simulink model "EE514test1"  (Simulink 7.6)
settings: Solver=ode45  StartTime=0.0  StopTime=10.0  RelTol=1e-6
undefined symbols (not defined in the file or in its folder): sigbuilder_block
settings Model: Creator=Nikola  LastModifiedBy=Nikola
settings DebuggingCC: StrictBusMsg=Warning
settings SimEventsCC: propDiagAttribOutput=1  propDiagFcnCallOutput=1  propDiagStatOutput=0

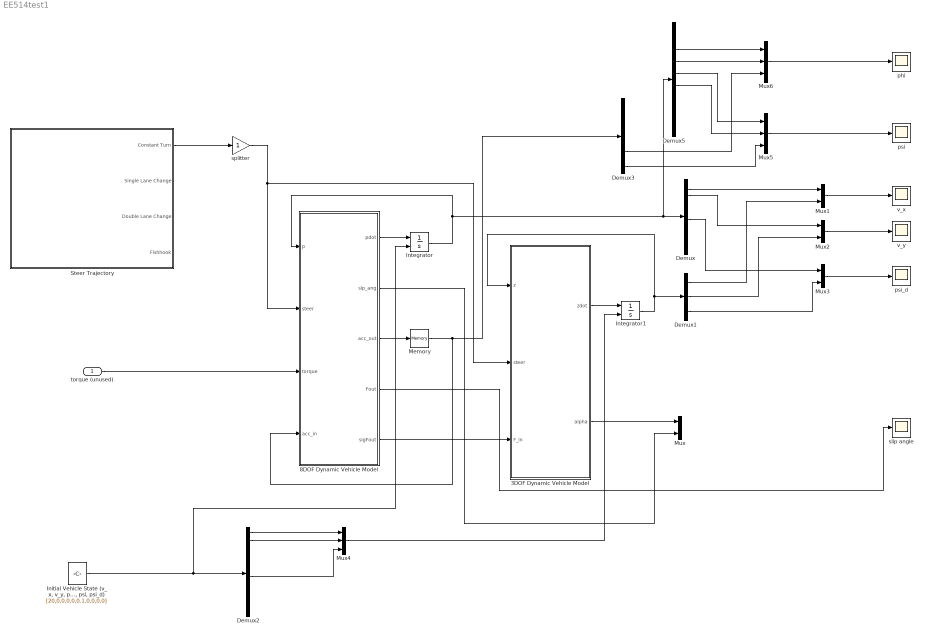
== system EE514test1 ==
  torque (unused) : Inport
  3DOF Dynamic Vehicle Model : Stateflow chart  TreatAsAtomicUnit=on
  8DOF Dynamic Vehicle Model : Stateflow chart  TreatAsAtomicUnit=on
  Demux : Demux  Outputs=10
  Demux1 : Demux  Outputs=3
  Demux2 : Demux  Outputs=10
  Demux3 : Demux  Outputs=5
  Demux5 : Demux  Outputs=10
  "Initial Vehicle State (v_x, v_y, phi, phi_d, psi, psi_d)" : Constant  Value=[20,0,0,0,0,0.1,0,0,0,0]
  Integrator : Integrator  InitialConditionSource=external  InitialCondition=[20,0,0,0,0,0,0,0,0,0]
  Integrator1 : Integrator  InitialConditionSource=external  InitialCondition=[20,0,0]
  Memory : Memory  X0=[0,0,0,0,0]  InheritSampleTime=on
  Mux{,1..3} (4 alike) : Mux  Inputs=2
  Mux4 : Mux  Inputs=3
  Mux5 : Mux  Inputs=3
  Mux6 : Mux  Inputs=3
  Steer Trajectory : Subsystem  Tag=STV Subsys  LoadFcn=sigbuilder_block('load');  StartFcn=sigbuilder_block('start');  StopFcn=sigbuilder_block('stop');  ClipboardFcn=sigbuilder_block('clipboard');  mask(Sigbuilder block){}
      mask help: Create and generate interchangeable groups of signals whose waveforms are piecewise linear.
      mask init:
      | if ~strcmp(get_param(bdroot(gcbh),'SimulationStatus'),'stopped') tuvar = sigbuilder_block('maskInit'); end
      settings: CopyFcn=sigbuilder_block('copy');  DeleteFcn=sigbuilder_block('delete');  ModelCloseFcn=sigbuilder_block('modelClose');  PreSaveFcn=sigbuilder_block('preSave');  NameChangeFcn=sigbuilder_block('namechange');  OpenFcn=sigbuilder_block('open',[-662.25 125.25 479.25 471.75 ]);  CloseFcn=sigbuilder_block('close');
      mask Display: plot(0,0,100,100,[10,10,40,40,10],[80,20,20,80,80],[40,10],[50,50], [40,27,10],[65,72,56],[40,25,25,10],[28,28,43,43]);
  phi : Scope
      settings: SaveName=ScopeData4
  psi : Scope
      settings: SaveName=ScopeData5
  psi_d : Scope
      settings: SaveName=ScopeData3
  slip angle : Scope
  splitter : Gain
  v_x : Scope
  v_y : Scope
      settings: SaveName=ScopeData2
  wires:
  torque (unused)/1 -> 8DOF Dynamic Vehicle Model/3(torque)
  8DOF Dynamic Vehicle Model/3(acc_out) -> Memory/1
  Memory/1 -> 8DOF Dynamic Vehicle Model/4(acc_in), Demux3/1
  8DOF Dynamic Vehicle Model/1(pdot) -> Integrator/1
  3DOF Dynamic Vehicle Model/1(zdot) -> Integrator1/1
  Integrator1/1 -> Demux1/1, 3DOF Dynamic Vehicle Model/1(z)
  splitter/1 -> 3DOF Dynamic Vehicle Model/2(steer), 8DOF Dynamic Vehicle Model/2(steer)
  3DOF Dynamic Vehicle Model/2(alpha) -> Mux/1
  8DOF Dynamic Vehicle Model/2(slp_ang) -> Mux/2
  Demux/1 -> Mux1/1
  Demux/2 -> Mux2/1
  Demux1/2 -> Mux2/2
  Demux/6 -> Mux3/1
  Mux1/1 -> v_x/1
  Mux3/1 -> psi_d/1
  Mux2/1 -> v_y/1
  Demux1/1 -> Mux1/2
  "Initial Vehicle State (v_x, v_y, phi, phi_d, psi, psi_d)"/1 -> Demux2/1, Integrator/2
  Demux2/1 -> Mux4/1
  Demux2/2 -> Mux4/2
  Demux2/6 -> Mux4/3
  Mux4/1 -> Integrator1/2
  Demux1/3 -> Mux3/2
  Integrator/1 -> 8DOF Dynamic Vehicle Model/1(p), Demux/1, Demux5/1
  Demux5/3 -> Mux6/1
  Demux5/4 -> Mux6/2
  Demux5/5 -> Mux5/1
  Demux5/6 -> Mux5/2
  Demux3/5 -> Mux5/3
  Demux3/4 -> Mux6/3
  Mux6/1 -> phi/1
  Mux5/1 -> psi/1
  8DOF Dynamic Vehicle Model/5(sigFout) -> 3DOF Dynamic Vehicle Model/3(F_in)
  8DOF Dynamic Vehicle Model/4(Fout) -> slip angle/1
  Steer Trajectory/1(Constant Turn) -> splitter/1

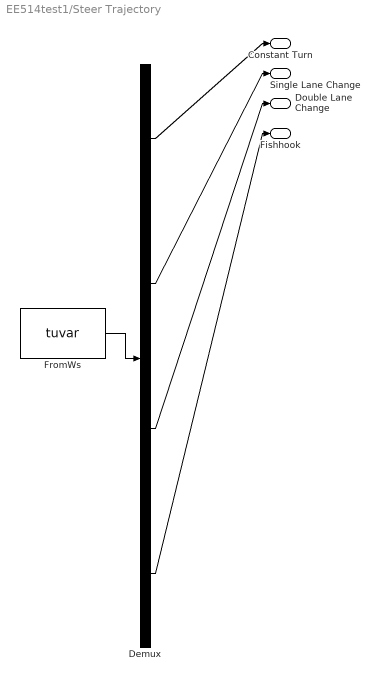
== system EE514test1/Steer Trajectory ==
  Demux : Demux  Tag=STV Demux
  FromWs : FromWorkspace  Tag=STV FromWs  VariableName=tuvar  SampleTime=0  SigBuilderData=DataTag0  VnvData=DataTag1
      SigBuilderData=|
      | common.afterFinalStr = 'Extrapolate'
      | common.sampleTime = 0
      | dataSet.timeRange = [0 10]
      | dataSet.name = 'Group 1'
      | sbobj.Groups.Name = 'Group 1'
      | sbobj.Groups.Signals(1).Name = 'Constant Turn'
      | sbobj.Groups.Signals(1).XData = [0 1 1.2 1.2 10]
      | sbobj.Groups.Signals(1).YData = [0 0 28 27.6 27.6]
      | sbobj.Groups.Signals(2).Name = 'Single Lane Change'
      | sbobj.Groups.Signals(2).XData = [0 1 1 1.2 1.2 1.4 1.4 10]
      | sbobj.Groups.Signals(2).YData = [0 0 10.05 10 -8.1 -8.1 0 0]
      | sbobj.Groups.Signals(3).Name = 'Double Lane Change'
      | sbobj.Groups.Signals(3).XData = [0 1 1 1.2 1.2 1.4 1.4 1.58 1.58 10]
      | sbobj.Groups.Signals(3).YData = [0 0 10 10 0 0 -11.4 -11.4 0 0]
      | sbobj.Groups.Signals(4).Name = 'Fishhook'
      | sbobj.Groups.Signals(4).XData = [0 1 1 1.2 1.2 1.45 1.45 10]
      | sbobj.Groups.Signals(4).YData = [0 0 15 15 -40 -40 0 0]
  Constant Turn : Outport  Tag=STV Outport
  Single Lane Change : Outport  Tag=STV Outport  Port=2
  Double Lane Change : Outport  Tag=STV Outport  Port=3
  Fishhook : Outport  Tag=STV Outport  Port=4
  wires:
  FromWs/1 -> Demux/1
  Demux/1 -> Constant Turn/1
  Demux/2 -> Single Lane Change/1
  Demux/3 -> Double Lane Change/1
  Demux/4 -> Fishhook/1

== matlab function 8DOF Dynamic Vehicle Model ==
  data: p input double; steer input double; pdot output double; torque input double; acc_in input double; slp_ang output double; acc_out output double; Fout output double; sigFout output double
function [pdot,slp_ang,acc_out,Fout,sigFout] = DVM8(p,steer,torque,acc_in)
 
%==output==%
pdot=zeros(10,1);
 
%==constants==%
g = 9.81; %m/s^2
%-------------%
 
%==current states==%
v_x = 1;
v_y = p(2);
phi = p(3);
phi_d = p(4);
psi = p(5);
psi_d = p(6);
 
a_x = acc_in(1);
a_y = acc_in(2);
phi_dd = acc_in(4);
psi_dd = acc_in(5);
%------------------%
 
%Car physical variables
l_fs = 1.01476;             %length from sprung mass CG to front suspension
l_rs = 1.67524;             %length from sprung mass CG to rear suspension
t_f = 1.540;                %front vehicle width
t_r = 1.530;                %rear vehicle width
h_f = 0.130;                %height from ground to front suspension
h_r = 0.110;                %height from ground to rear suspension
h_cgs = 0.567851;           %height from ground to sprung CG
h_cguf = 0.320;             %height from ground to front unsprung CG
h_cgur = 0.320;             %height from ground to rear unsprung CG
M = 1704.7;                 %total vehicle mass
M_uf = 98.1;                %unsprung front mass
M_ur = 79.7;                %unsprung rear mass
I_xxs = 440.911;            %sprung XX inertia
I_xys = 0;                  %sprung XY inertia
I_xzs = 7.54097;            %sprung XZ inertia
I_yys = 2498.900;           %sprung YY inertia
I_yzs = 0;                  %sprung yz inertia
I_zzs = 2619.28;            %sprung ZZ inertia
I_zzuf = M_uf*(t_f/2)^2;    %front unsprung ZZ inertia
I_zzur = M_ur*(t_r/2)^2;    %rear unsprung ZZ inertia
I_tlf = 0.99;               %front left tire inertia
I_trf = 0.99;               %front right tire inertia
I_tlr = 0.99;               %rear left tire inertia
I_trr = 0.99;               %rear right tire inertia
 
%spring/dampers
K_spf = 27.85; %N/mm
K_spr = 18.16; %N/mm
 
B_f = 2.9915; %N-s/mm
B_r = 2.9915; %N-s/mm
 
%anti_roll bars
K_rf = 384.0*180/pi; %Nm/rad
K_rr = 344.4*180/pi;
 
%roll stiffness
K_phif = 0.766*K_spf*1000*t_f^2/2 + K_rf;%
K_phir = 0.827*K_spr*1000*t_r^2/2 + K_rr;%
K_phi = (K_phif + K_phir);
 
%roll damping
B_phif = 0.766*B_f*1000*t_f^2/2; %Nm-s/rad
B_phir = 0.827*B_r*1000*t_r^2/2;
B_phi = (B_phif + B_phir);
 
K_sr = 15.97; %steering-to-wheel angle ratio
 
%==calculated parameters==%
L = l_fs + l_rs;                    %distance from front to rear suspension
M_s = M - M_uf - M_ur;              %sprung mass
l_cgs = (M_ur*l_rs - M_uf*l_fs)/M;  %distance from vehicle CG to sprung CG
l_f = l_fs + l_cgs;                 %distance from vehicle CG to front suspension
l_r = l_rs - l_cgs;                 %distance from vehicle CG to rear suspension
M_f = M*l_r/L;                      %front vehicle mass
M_r = M*l_f/L;                      %rear vehicle mass
h_o = h_f + l_f*(h_r - h_f)/L;      %height from ground to roll axis
h_s = h_cgs - h_o;                  %height from roll axis to sprung CG
h_uf = h_cguf - h_o;                %height from roll axis to front suspension
h_ur = h_cgur - h_o;                %height from roll axis to rear suspension
h_cg = (M_s*h_cgs + M_uf*h_cguf + M_ur*h_cgur)/M;   %height from gound to vehicle CG
%----------------------------%
 
%==tire properties==%
varx = [...
    0.0, 0.0;...
    0.1, 0.6;...
    0.15, 0.85;...
    1.0, 0.4]; %slip curve coordinates (slip-%, mu)
vary = [...
    0.0, 0.0;...
    0.08, 0.4;...
    0.15, 0.6;...
    0.3, 0.8;...
    1.0, 0.4]; %slip curve coordinates (slip-%, mu) 
varM = [...
    0.0, 0.0;...
    0.1, 0.0005;...
    0.3, 0.00025;...
    1.0, 0.0]; %slip angle (slip-angle, Moment-arm)
 
 
%tire properties
t_wid = 0.175;
t_rad = 0.292;
t_pressure = 275000;
 
%---------------------%
 
%==steering inputs==%
d_steer = steer;
%-------------------%
 
%==calculate internal accelerations==%
a_sx = a_x ...
     - psi_d*v_y ...
     - 2*h_s*phi_d*psi_d*cos(phi) ...
     - l_cgs*psi_d^2;
a_sy = psi_d*v_x ...
     + l_cgs*psi_dd ...
     + h_s*cos(phi)*phi_dd ...
     - h_s*phi_d^2*sin(phi) ...
     - h_s*psi_d^2*sin(phi);
a_ufx = a_x - l_f*psi_d^2;
a_ufy = a_y + l_f*psi_dd;
a_urx = a_x + l_r*psi_d^2;
a_ury = a_y - l_r*psi_dd;
%-------------------------------------%
 
%==rotation Matrix==%
ROT = [1,0,0;
       0,cos(phi),sin(phi);
       0,-sin(phi),cos(phi)];
 
I_b = [I_xxs+M_s*h_s^2,I_xys,I_xzs+M_s*h_s*l_cgs;...
       I_xys,I_yys+M_s*(h_s^2+l_cgs^2),I_yzs;...
       I_xzs+M_s*h_s*l_cgs,I_yzs,I_zzs+M_s*l_cgs^2];
   
I_c = ROT*I_b*ROT'; %chassis M.o.I. tensor
 
I_zzus = M_uf*l_f^2 + ...
         M_ur*l_r^2 + ...
         I_zzuf + I_zzur;
 
I_xxo = I_c(1,1);
I_zzo = I_c(3,3) + I_zzus; %effective I_zz
%---------------------------------------------%
 
%==Dynamic Weight Transfer Forces==%
Fzax = (M_s*h_s*a_sx + M_uf*h_uf*a_ufx + M_ur*h_ur*a_urx)/(2*L);
Fzayf = 1/t_f*(M_s*l_r*h_f/L*a_sy + M_uf*h_uf*a_ufy);
Fzayr = 1/t_r*(M_s*l_f*h_r/L*a_sy + M_ur*h_ur*a_ury);
Fzphif = -1/t_f*(K_phif*phi + B_phif*phi_d);
Fzphir = -1/t_r*(K_phir*phi + B_phir*phi_d);
%----------------------------------%
 
%==Tire Normal Forces==% 
Fzlf = M*g*l_r/(2*L) - Fzax - Fzayf + Fzphif;
Fzrf = M*g*l_r/(2*L) - Fzax + Fzayf - Fzphif;
Fzlr = M*g*l_f/(2*L) + Fzax - Fzayr + Fzphir;
Fzrr = M*g*l_f/(2*L) + Fzax + Fzayr - Fzphir;
%----------------------%
 
%==Tire Longitudinal/Lateral Forces==%
 
%left front wheel velocity
v_xlf = v_x + psi_d*t_f/2;
v_ylf = v_y + psi_d*l_f;
 
%right front wheel velocity
v_xrf = v_x - psi_d*t_f/2;
v_yrf = v_y + psi_d*l_f;
 
%left rear wheel velocity
v_xlr = v_x + psi_d*t_r/2;
v_ylr = v_y - psi_d*l_r;
 
%right rear wheel velocity
v_xrr = v_x - psi_d*t_r/2;
v_yrr = v_y - psi_d*l_r;
 
%tire updates
omega_lf = (v_xlf^2 + v_ylf^2)^(1/2);
omega_rf = (v_xrf^2 + v_yrf^2)^(1/2);
omega_lr = (v_xlr^2 + v_ylr^2)^(1/2);
omega_rr = (v_xrr^2 + v_yrr^2)^(1/2);
 
%==Linear Cruise Control=%
if v_x < 11.1
    if omega_lf > omega_rf
        Mtlf = (11.1 - v_x)*200;
        Mtrf = 0;
    else
        Mtlf = 0;
        Mtrf = (11.1 - v_x)*200;
    end
else
    Mtlf = 0;
    Mtrf = 0;
end

%The tire moments are unused...
Mtlf = 0;
Mtrf = 0;
Mtlr = 0;
Mtrr = 0;
%-------------------------%
 
%get steering angle
delta = d_steer/(180*K_sr)*pi; %radians
beta = atan(v_y/v_x);
beta_lf = atan(v_ylf/v_xlf);
beta_rf = atan(v_yrf/v_xrf);
beta_lr = atan(v_ylr/v_xlr);
beta_rr = atan(v_yrr/v_xrr);
 
%Interpolate forces
%Linearized Force Coefficients (C_alpha)
C_alf = vary(2,2)/vary(2,1)*Fzlf;
C_arf = vary(2,2)/vary(2,1)*Fzrf;
C_alr = vary(2,2)/vary(2,1)*Fzlr;
C_arr = vary(2,2)/vary(2,1)*Fzrr;
 
a_lf = beta_lf - delta;
a_rf = beta_rf - delta;
a_lr = beta_lr;
a_rr = beta_rr;
 
slp_ang = [C_alf,C_arf,C_alr,C_arr];
 
%Linear Cruise Control for constant v_x
if v_x < 11.1
    Fxtf = (11.1-v_x)*20000;
else
    Fxtf = 0; %no torque
end
 
Fxtlf = 0;
Fxtrf = 0;
Fxtlr = 0;
Fxtrr = 0;
 
Fytlf = -a_lf*C_alf;
Fytrf = -a_rf*C_arf;
Fytlr = -a_lr*C_alr;
Fytrr = -a_rr*C_arr;
 
 
Fxlf = Fxtlf*cos(delta) - Fytlf*sin(delta);
Fxrf = Fxtrf*cos(delta) - Fytrf*sin(delta);
Fxlr = Fxtlr;
Fxrr = Fxtrr;
 
Fylf = Fytlf*cos(delta) + Fxtlf*sin(delta);
Fyrf = Fytrf*cos(delta) + Fxtrf*sin(delta);
Fylr = Fytlr;
Fyrr = Fytrr;
 
Fout = [Fytlf,Fytrf,Fytlr,Fytrr];


%The tire moments are unused here...
Mzlf = 0;
Mzrf = 0;
Mzlr = 0;
Mzrr = 0;
%---------------------------------------%
 
%Omeaga/Alpha of Wheels
alpha_lf_new = (Fxtlf*t_rad + Mtlf)/I_tlf;
alpha_rf_new = (Fxtrf*t_rad + Mtrf)/I_trf;
alpha_lr_new = (Fxtlr*t_rad + Mtlr)/I_tlr;
alpha_rr_new = (Fxtrr*t_rad + Mtrr)/I_trr;
 
% alpha_lf_new = 0;
% alpha_rf_new = 0;
% alpha_lr_new = 0;
% alpha_rr_new = 0;
 
 
%==Torques==%
T_phif = -K_phif*phi - B_phif*phi_d;
T_phir = -K_phir*phi - B_phir*phi_d;
%-----------%
 
%==Sum forces and torques==%
sigFx = Fxlf + Fxrf + Fxlr + Fxrr;
sigFy = Fylf + Fyrf + Fylr + Fyrr;
sigTxs = T_phif + T_phir - ...
         M_s*g*h_s*sin(phi) + M_s*h_s*a_sy*cos(phi);
sigTz = (Fylf + Fyrf)*l_f - (Fylr + Fyrr)*l_r + ...
        t_f/2*(Fxlf - Fxrf) + t_r/2*(Fxlr - Fxrr) + ...
        Mzlf + Mzrf + Mzlr + Mzrr;

sigFout = [sigFx, sigFy, sigTxs, sigTz];    
    
%--------------------------%
 
%==Update independent variables==%
a_x_new = (sigFx + ...
           M_s.*(-2*h_s.*phi_d.*psi_d.*cos(phi) - ... 
           h_s.*psi_dd.*sin(phi)))./M;
a_y_new = (sigFy - ...
           M_s*(-h_s*phi_dd*cos(phi) + ...
           h_s*phi_d^2*sin(phi) + ...
           h_s*psi_d^2*sin(phi)))./M;
phi_dd_new = (sigTxs - ...
           (I_xzs+M_s*h_s*l_cgs)*cos(phi)*psi_dd + ...
           (I_xzs+M_s*h_s*l_cgs)*sin(phi)*phi_d*psi_d + ...
           (I_zzs - I_yys - M_s*h_s^2)*sin(phi)*cos(phi)*psi_d^2)./ ...
           (I_xxs+M_s*h_s^2);
psi_dd_new = (sigTz - ...
           (I_xzs+M_s*h_s*l_cgs)*cos(phi)*phi_dd - ...
           (I_xzs+M_s*h_s*l_cgs)*sin(phi)*phi_d^2 - ...
            M_s*h_s*a_x*sin(phi) - ...
           (I_zzs - I_yys - M_s*h_s^2)*sin(phi)*cos(phi)*psi_d*phi_d)./ ...
            I_zzo;
 
%acceleration outputs
acc_out = [a_x_new,a_y_new,a_sy,phi_dd_new,psi_dd_new];        
        
%X
pdot(1) = a_x_new;
%Y   
pdot(2) = a_y_new;
%PHI
pdot(3) = phi_d;
pdot(4) = phi_dd_new;
%PSI
pdot(5) = psi_d;
pdot(6) = psi_dd_new;
%WHEELS
pdot(7) = alpha_lf_new;
pdot(8) = alpha_rf_new;
pdot(9) = alpha_lr_new;
pdot(10) = alpha_rr_new;
%SPRUNG BODY
%----------------------------------%
%end
%nd
%d
%

== matlab function 3DOF Dynamic Vehicle Model ==
  data: z input double; steer input double; zdot output double; F_in input double; alpha output double
function [zdot,alpha] =  DVM3(z, steer, F_in)

%Inputs
v_x = z(1);
v_y = z(2);
psi_d = z(3);

F_x = F_in(1);
F_y = F_in(2);
T_z = F_in(3);

%Car physical variables
M = 1704.7;                 %total vehicle mass
l_fs = 1.01476;             %length from CG to front suspension
I_zzs = 2619.28;            %sprung ZZ inertia
K_sr = 15.97;               %steering-to-wheel angle ratio
C_af = 25730;               %Lateral Slip Stiffness

%Slip Angle
delta = steer/(180*K_sr)*pi;
beta = atan(v_y/v_x);

alpha = beta-delta;

%Tire Forces
F_xt = 0;
F_yt = -C_af*alpha;

%F_x = -F_yt*sin(delta);
%F_y = F_yt*cos(delta);
%T_z = -l_fs*C_af*cos(alpha);

%State Output
a_x = (1/M)*(v_y*psi_d+F_x);
a_y = (1/M)*(-v_x*psi_d+F_y);
psi_dd = (1/I_zzs)*(T_z);

zdot = [a_x, a_y, psi_dd];

%----------------------------------%
%end
